simulink subsystem "noiseFilter"  (R2026a)
settings: Solver=VariableStepAuto
settings Model: Creator=maxhu  LastModifiedBy=maxhu

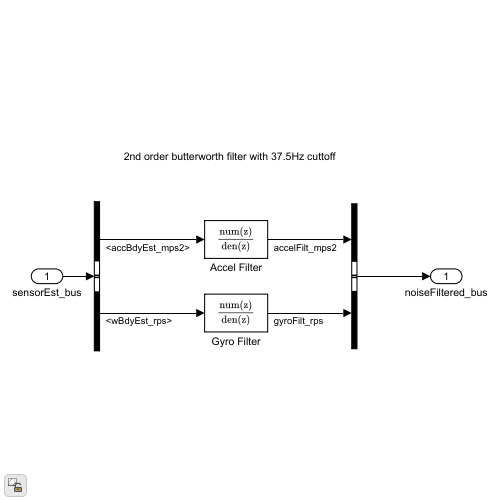
[thumbnail: Simulink's stored preview of the top-level diagram]
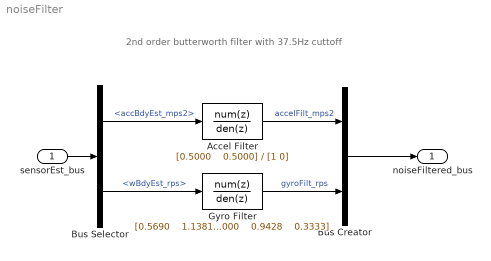
== system noiseFilter ==
  note: 2nd order butterworth filter with 37.5Hz cuttoff
  sensorEst_bus : Inport
  Accel Filter : DiscreteTransferFcn  Numerator="[0.5000    0.5000]"  Denominator=[1 0]
  Bus Creator : BusCreator  Inputs=2
  Bus Selector : BusSelector  OutputSignals=accBdyEst_mps2,wBdyEst_rps
  Gyro Filter : DiscreteTransferFcn  Numerator="[0.5690    1.1381    0.5690]"  Denominator="[1.0000    0.9428    0.3333]"
  noiseFiltered_bus : Outport
  wires:
  sensorEst_bus/1 -> Bus Selector/1
  Bus Creator/1 -> noiseFiltered_bus/1
  Bus Selector/2 -> Gyro Filter/1  "<wBdyEst_rps>"
  Gyro Filter/1 -> Bus Creator/2  "gyroFilt_rps"
  Accel Filter/1 -> Bus Creator/1  "accelFilt_mps2"
  Bus Selector/1 -> Accel Filter/1  "<accBdyEst_mps2>"
